simulink model "sim_Start_2021b"  (R2023a)
settings: Solver=FixedStepDiscrete  StartTime=0.0  StopTime=30  FixedStep=0.01  RelTol=1e-3
undefined symbols (not defined in the file or in its folder): InputPWM, WheelSpeed
libraries: mobileRoboticsTrainingLib x7
settings Model: Creator=Boitumelo  LastModifiedBy=josephstewart
settings DebuggingCC: UnconnectedInputMsg=warning  UnconnectedOutputMsg=warning  UnconnectedLineMsg=warning
settings ModelReferenceCC: EnableRefExpFcnMdlSchedulingChecks=on
settings RTWCC: DLArmComputeVersion=19.05

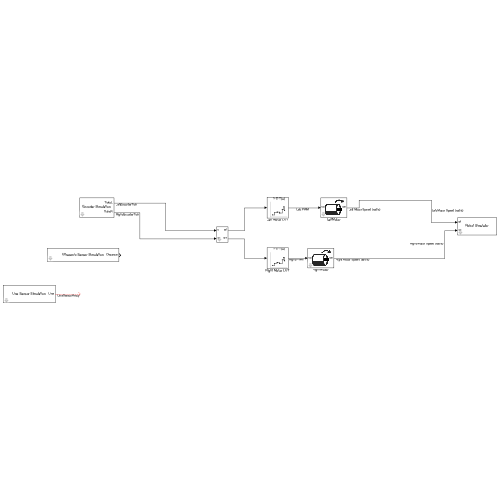
[thumbnail: Simulink's stored preview of the top-level diagram]
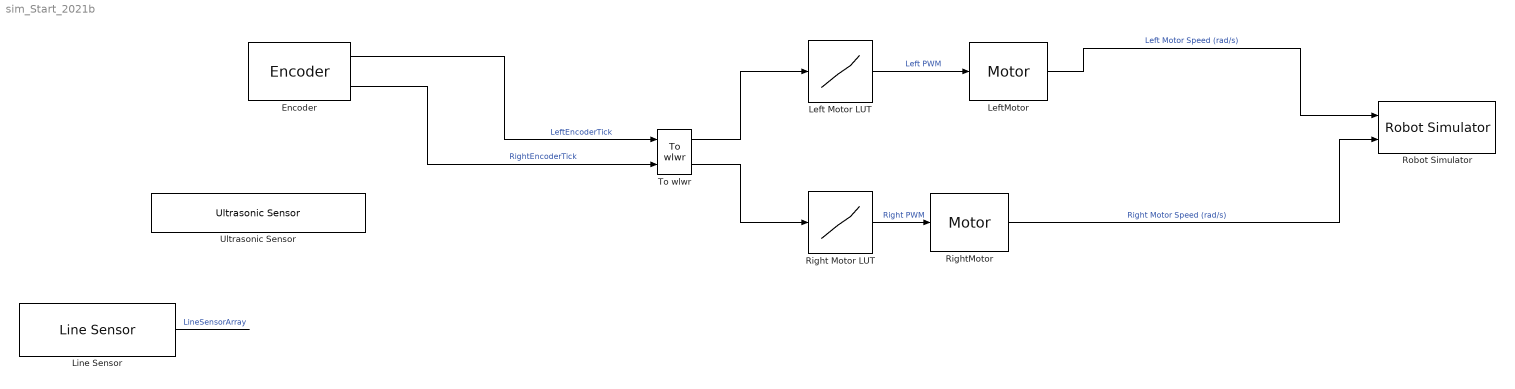
== system sim_Start_2021b ==
  Encoder : mobileRoboticsTrainingLib/Encoder  axleLength=axleLength  wheelR=wheelR  ticksPerRot=ticksPerRot
      settings: SourceProductName=Mobile Robotics Training Library
  Left Motor LUT : Lookup_n-D  NumberOfTableDimensions=1  BreakpointsForDimension1=WheelSpeed  Table=InputPWM  InterpMethod=Nearest  ExtrapMethod=Clip  InternalRulePriority=Speed  RndMeth=Simplest
  LeftMotor : mobileRoboticsTrainingLib/Motor  motorPlant=wheelMotorModel  sensorType=Speed
      settings: SourceProductName=Mobile Robotics Training Library
  Line Sensor : mobileRoboticsTrainingLib/Line Sensor  mapVariable=mapForSim  envVal=1  lineVal=0  sensOff=[0 0; 0 0; 0 0; 0 0]
      settings: SourceProductName=Mobile Robotics Training Library
  Right Motor LUT : Lookup_n-D  NumberOfTableDimensions=1  BreakpointsForDimension1=WheelSpeed  Table=InputPWM  InterpMethod=Nearest  ExtrapMethod=Clip  InternalRulePriority=Speed  RndMeth=Simplest
  RightMotor : mobileRoboticsTrainingLib/Motor  motorPlant=wheelMotorModel  sensorType=Speed
      settings: SourceProductName=Mobile Robotics Training Library
  Robot Simulator : mobileRoboticsTrainingLib/Robot Simulator  Priority=99  mapVar=mapForSim  startX=0.2  startY=0  startTheta=90  axleLength=axleLength  wheelR=wheelR
  To wlwr : mobileRoboticsTrainingLib/To wlwr  axleLength=axleLength  wheelR=wheelR
  Ultrasonic Sensor : mobileRoboticsTrainingLib/Ultrasonic Sensor  mapVar=mapForSim  maxSenRange=2  minSenRange=0.02  senRes=0.01  sensOff=[0 0]
      link override Look up Distance Value/Subsystem/Look up Sensor Value/Lookup Obstacle Map/Direct Lookup Table (n-D): TableIsInput=off
      settings: SourceProductName=Mobile Robotics Training Library
  wires:
  Right Motor LUT/1 -> RightMotor/1  "Right PWM"
  Left Motor LUT/1 -> LeftMotor/1  "Left PWM"
  Encoder/1 -> To wlwr/1  "LeftEncoderTick"
  Encoder/2 -> To wlwr/2  "RightEncoderTick"
  To wlwr/1 -> Left Motor LUT/1
  To wlwr/2 -> Right Motor LUT/1
  Line Sensor/1 -> ?  "LineSensorArray"
  RightMotor/1 -> Robot Simulator/2  "Right Motor Speed (rad/s)"
  LeftMotor/1 -> Robot Simulator/1  "Left Motor Speed (rad/s)"
